simulink model "Sim_con_AWU"  (R2023b)
settings: Solver=VariableStepAuto  StartTime=0.0  StopTime=10.0  RelTol=1e-3
values from neighbouring files (symbols this model uses):
  bat_awu_den = [k_bat_inf zero_battery_current*k_bat_inf]    [Variables.m]
  bat_awu_num = -zero_battery_current    (= -916)    [Variables.m]
  cell_awu_den = [k_cell_inf zero_cell_current*k_cell_inf]    [Variables.m]
  cell_awu_num = -zero_cell_current    (= -2.33)    [Variables.m]
  k_bat_inf = K_battery_current    (= 6.415)    [Variables.m]
  k_cell_inf = K_cell_current    (= 13.69)    [Variables.m]
settings Model: Creator=Admin  LastModifiedBy=gonza
settings ModelReferenceCC: EnableRefExpFcnMdlSchedulingChecks=on

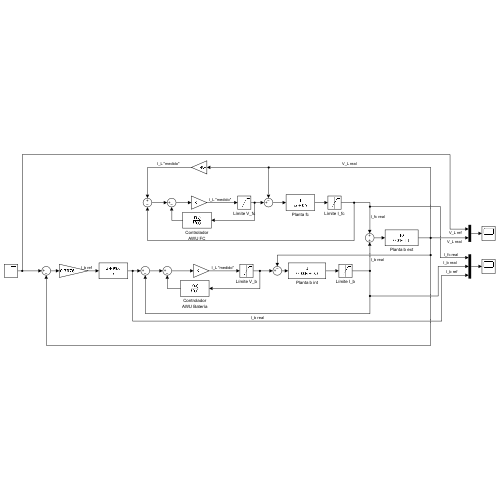
[thumbnail: Simulink's stored preview of the top-level diagram]
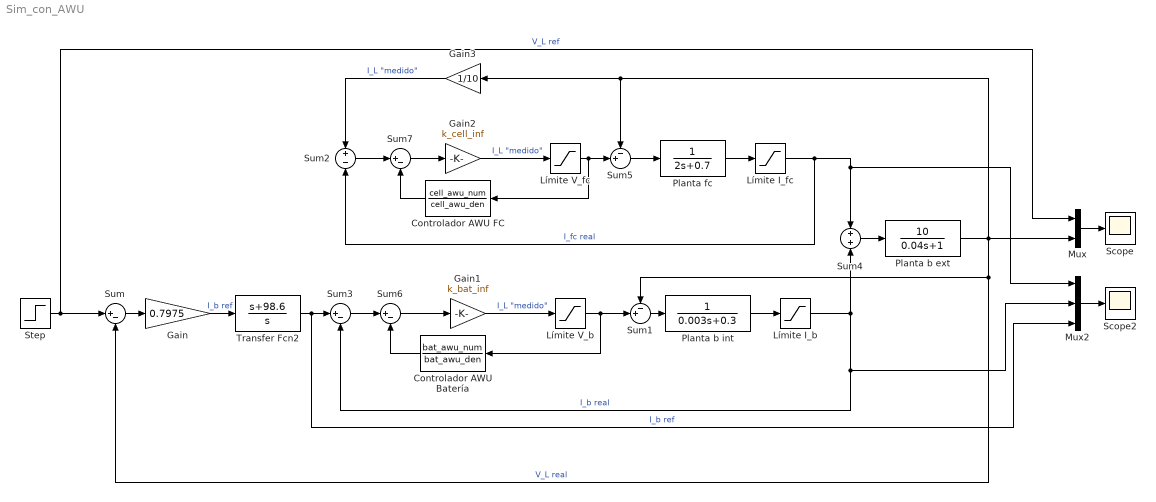
== system Sim_con_AWU ==
  Controlador AWU Batería : TransferFcn  Numerator=bat_awu_num  Denominator=bat_awu_den
  Controlador AWU FC : TransferFcn  Numerator=cell_awu_num  Denominator=cell_awu_den
  Gain : Gain  Gain=0.7975
  Gain1 : Gain  Gain=k_bat_inf
  Gain2 : Gain  Gain=k_cell_inf
  Gain3 : Gain  Gain=1/10
  Límite I_b : Saturate  UpperLimit=120  LowerLimit=-120
  Límite I_fc : Saturate  UpperLimit=200  LowerLimit=0
  Límite V_b : Saturate  UpperLimit=400  LowerLimit=-400
  Límite V_fc : Saturate  UpperLimit=450  LowerLimit=0
  Mux : Mux  Inputs=2
  Mux2 : Mux  Inputs=3
  Planta b ext : TransferFcn  Numerator=[10]  Denominator=[0.04 1]
  Planta b int : TransferFcn  Denominator=[0.003 0.3]
  Planta fc : TransferFcn  Denominator=[2 0.7]
  Scope : Scope
  Scope2 : Scope
  Step : Step  After=250  SampleTime=0
  Sum{,3,6..7} (4 alike) : Sum  Inputs=|+-
  Sum1 : Sum  Inputs=-+|
  Sum2 : Sum  Inputs=+|-
  Sum4 : Sum  Inputs=+|+
  Sum5 : Sum  Inputs=-+|
  Transfer Fcn2 : TransferFcn  Numerator=[1 98.6]  Denominator=[1 0]
  wires:
  Step/1 -> Sum/1, Mux/1  "V_L ref"
  Transfer Fcn2/1 -> Mux2/3, Sum3/1  "I_b ref"
  Sum4/1 -> Planta b ext/1
  Planta b ext/1 -> Sum5/1, Gain3/1, Mux/2, Sum1/1, Sum/2  "V_L real"
  Mux/1 -> Scope/1
  Límite I_b/1 -> Sum3/2, Mux2/2, Sum4/2  "I_b real"
  Límite I_fc/1 -> Mux2/1, Sum4/1, Sum2/2  "I_fc real"
  Planta b int/1 -> Límite I_b/1
  Planta fc/1 -> Límite I_fc/1
  Gain3/1 -> Sum2/1  "I_L \"medido\""
  Límite V_b/1 -> Controlador AWU Batería/1, Sum1/2
  Sum1/1 -> Planta b int/1
  Límite V_fc/1 -> Controlador AWU FC/1, Sum5/2
  Sum5/1 -> Planta fc/1
  Mux2/1 -> Scope2/1
  Sum6/1 -> Gain1/1
  Controlador AWU Batería/1 -> Sum6/2
  Gain1/1 -> Límite V_b/1  "I_L \"medido\""
  Sum3/1 -> Sum6/1
  Controlador AWU FC/1 -> Sum7/2
  Sum7/1 -> Gain2/1
  Gain2/1 -> Límite V_fc/1  "I_L \"medido\""
  Sum2/1 -> Sum7/1
  Sum/1 -> Gain/1
  Gain/1 -> Transfer Fcn2/1  "I_b ref"
